simulink model "Hybrid_PID"  (R2016a)
settings: Solver=ode4  StartTime=0.0  StopTime=inf  FixedStep=ts  RelTol=1e-3
values from neighbouring files (symbols this model uses):
  db_x = 0.5    [center_and_move.m]
  db_y = 2    [center_and_move.m]
  db_z = 0.001    [center_and_move.m]
  fpos = -z_net    [center_and_move.m]
  kdx = 1.2    [center_and_move.m]
  kdy = 4    [center_and_move.m]
  kdz = 0.55    [center_and_move.m]
  kix = 3.5    [center_and_move.m]
  kiy = 1.9    [center_and_move.m]
  kiz = 10    [center_and_move.m]
  kpx = 85    [center_and_move.m]
  kpy = 485    [center_and_move.m]
  kpz = 2.5    [center_and_move.m]
  ts = 0.001    [center_and_move.m]
  tsim = 25    [center_and_move.m]
  xpos = -x_net    [center_and_move.m]    (also in genScanMatrix.m = x_net2)
  ypos = -y_net    [center_and_move.m]    (also in genScanMatrix.m = y_net)
  zpos = z_net    [genScanMatrix.m]
undefined symbols (not defined in the file or in its folder): amp, bias, f
libraries: slrtlib x11, dspswit3 x7, xpcmeasurementcomputinglib x5, simulink_extras x3, simulink x3, xpcconteclib x3, xpcutilitieslib x1, xpcrtudplib x1
settings Model: SimulationMode=external  Creator=Biorobotics  LastModifiedBy=Biorobotics
settings SolverCC: EnableConcurrentExecution=on
settings DataIOCC: SaveFormat=StructureWithTime
settings OptimizationCC: BlockReduction=off  OptimizeBlockIOStorage=off  BufferReuse=off  GlobalBufferReuse=off  ExpressionFolding=off  LocalBlockOutputs=off
settings HardwareCC: ProdBitPerPointer=32  ProdLargestAtomicFloat=None  ProdWordSize=32  ProdLongLongMode=on  ProdHWDeviceType=Generic->32-bit x86 compatible
settings RTWCC: SystemTargetFile=slrt.tlc  TemplateMakefile=slrt_default_tmf  Description=Simulink Real-Time  RTWCompilerOptimization=on

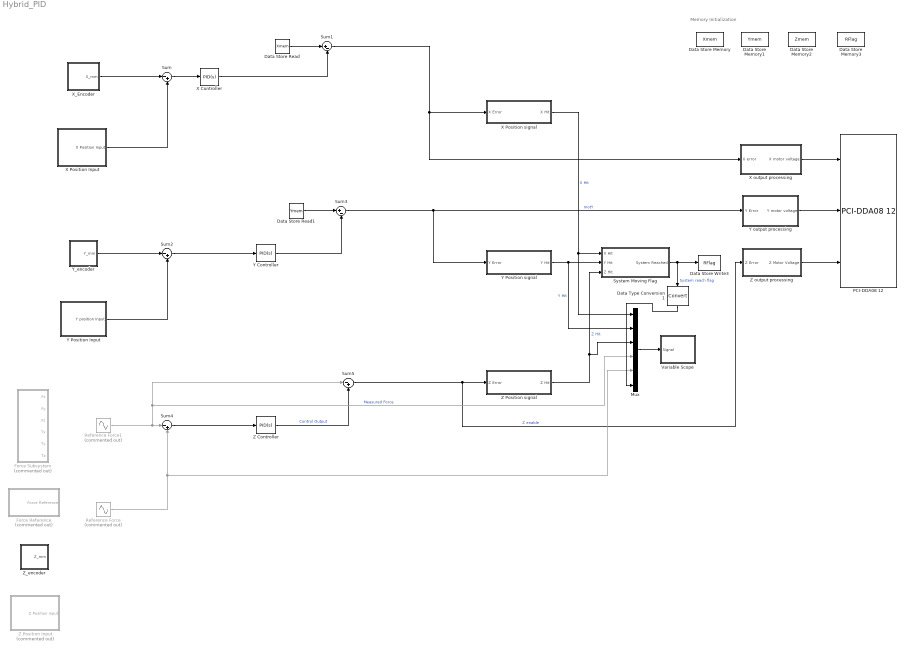
== system Hybrid_PID ==
  note: Memory Initialization
  Data Store Memory : DataStoreMemory  DataStoreName=Xmem  ReadBeforeWriteMsg=warning  WriteAfterWriteMsg=warning  WriteAfterReadMsg=warning  ShowAdditionalParam=off
  Data Store Memory1 : DataStoreMemory  DataStoreName=Ymem  ReadBeforeWriteMsg=warning  WriteAfterWriteMsg=warning  WriteAfterReadMsg=warning  ShowAdditionalParam=off
  Data Store Memory2 : DataStoreMemory  DataStoreName=Zmem  ReadBeforeWriteMsg=warning  WriteAfterWriteMsg=warning  WriteAfterReadMsg=warning  ShowAdditionalParam=off
  Data Store Memory3 : DataStoreMemory  DataStoreName=RFlag  ReadBeforeWriteMsg=warning  WriteAfterWriteMsg=warning  WriteAfterReadMsg=warning  ShowAdditionalParam=off
  Data Store Read : DataStoreRead  DataStoreName=Xmem
  Data Store Read1 : DataStoreRead  DataStoreName=Ymem
  Data Store Write3 : DataStoreWrite  DataStoreName=RFlag
  Data Type Conversion1 : DataTypeConversion
  Force Reference : Subsystem  Commented=on
  Force Subsystem : Subsystem  Commented=on
  Mux : Mux  Inputs=6
  "PCI-DDA08 12 " : xpcmeasurementcomputinglib/D//A/PCI-DDA08 12   channel=[1 2 3]  range=[-10 -10 -10]  reset=[1]  initValue=[0]  sampletime=ts  pci_dev=-1
  Reference Force : Sin  Commented=on  Amplitude=amp  Bias=bias  Frequency=f*2*pi  SampleTime=ts
  Reference Force1 : Sin  Commented=on  Amplitude=amp  Bias=bias  Frequency=f*2*pi  SampleTime=ts
  Sum{,2,4..5} (4 alike) : Sum  Inputs=|-+
  Sum1 : Sum  Inputs=|+-
  Sum3 : Sum  Inputs=|+-
  System Moving Flag : Subsystem
  Variable Scope : Subsystem
  X Controller : simulink/Continuous/PID Controller  Controller=PID  TimeDomain=Continuous-time  SampleTime=-1  IntegratorMethod=Forward Euler  FilterMethod=Forward Euler  Form=Parallel  UseFilter=on  ControllerParametersSource=internal  P=kpx  I=kix  D=kdx  N=100  InitialConditionSource=internal  InitialConditionForIntegrator=0  InitialConditionForFilter=0  ExternalReset=none  ZeroCross=off  LimitOutput=off  UpperSaturationLimit=inf  LowerSaturationLimit=-inf  LinearizeAsGain=on  AntiWindupMode=none  Kb=1  TrackingMode=off  Kt=1  PParamMin=[]  PParamMax=[]  IParamMin=[]  IParamMax=[]  DParamMin=[]  DParamMax=[]  NParamMin=[]  NParamMax=[]  KbParamMin=[]  KbParamMax=[]  KtParamMin=[]  KtParamMax=[]  POutMin=[]  POutMax=[]  IOutMin=[]  IOutMax=[]  DOutMin=[]  DOutMax=[]  NOutMin=[]  NOutMax=[]  KbOutMin=[]  KbOutMax=[]  KtOutMin=[]  KtOutMax=[]  IntegratorOutMin=[]  IntegratorOutMax=[]  FilterOutMin=[]  FilterOutMax=[]  SumOutMin=[]  SumOutMax=[]  SumI1OutMin=[]  SumI1OutMax=[]  SumI2OutMin=[]  SumI2OutMax=[]  SumI3OutMin=[]  SumI3OutMax=[]  SumDOutMin=[]  SumDOutMax=[]  SaturationOutMin=[]  SaturationOutMax=[]  IntegratorContinuousStateAttributes=''  IntegratorStateMustResolveToSignalObject=off  IntegratorRTWStateStorageClass=Auto  FilterContinuousStateAttributes=''  FilterStateMustResolveToSignalObject=off  FilterRTWStateStorageClass=Auto  DifferentiatorICPrevScaledInput=0  DifferentiatorOutMin=[]  DifferentiatorOutMax=[]
  X Position Input : Subsystem
  X Position signal : Subsystem
  X output processing : Subsystem
  X_Encoder : Subsystem
  Y Controller : simulink/Continuous/PID Controller  Controller=PID  TimeDomain=Continuous-time  SampleTime=-1  IntegratorMethod=Forward Euler  FilterMethod=Forward Euler  Form=Parallel  UseFilter=on  ControllerParametersSource=internal  P=kpy  I=kiy  D=kdy  N=100  InitialConditionSource=internal  InitialConditionForIntegrator=0  InitialConditionForFilter=0  ExternalReset=none  LimitOutput=off  UpperSaturationLimit=inf  LowerSaturationLimit=-inf  LinearizeAsGain=on  AntiWindupMode=none  Kb=1  TrackingMode=off  Kt=1  PParamMin=[]  PParamMax=[]  IParamMin=[]  IParamMax=[]  DParamMin=[]  DParamMax=[]  NParamMin=[]  NParamMax=[]  KbParamMin=[]  KbParamMax=[]  KtParamMin=[]  KtParamMax=[]  POutMin=[]  POutMax=[]  IOutMin=[]  IOutMax=[]  DOutMin=[]  DOutMax=[]  NOutMin=[]  NOutMax=[]  KbOutMin=[]  KbOutMax=[]  KtOutMin=[]  KtOutMax=[]  IntegratorOutMin=[]  IntegratorOutMax=[]  FilterOutMin=[]  FilterOutMax=[]  SumOutMin=[]  SumOutMax=[]  SumI1OutMin=[]  SumI1OutMax=[]  SumI2OutMin=[]  SumI2OutMax=[]  SumI3OutMin=[]  SumI3OutMax=[]  SumDOutMin=[]  SumDOutMax=[]  SaturationOutMin=[]  SaturationOutMax=[]  IntegratorContinuousStateAttributes=''  IntegratorStateMustResolveToSignalObject=off  IntegratorRTWStateStorageClass=Auto  FilterContinuousStateAttributes=''  FilterStateMustResolveToSignalObject=off  FilterRTWStateStorageClass=Auto  DifferentiatorICPrevScaledInput=0  DifferentiatorOutMin=[]  DifferentiatorOutMax=[]
  Y Position Input : Subsystem
  Y Position signal : Subsystem
  Y output processing : Subsystem
  "Y_encoder " : Subsystem
  Z Controller : simulink/Continuous/PID Controller  Controller=PID  TimeDomain=Continuous-time  SampleTime=-1  IntegratorMethod=Forward Euler  FilterMethod=Forward Euler  Form=Parallel  UseFilter=on  ControllerParametersSource=internal  P=kpz  I=kiz  D=kdz  N=100  InitialConditionSource=internal  InitialConditionForIntegrator=0  InitialConditionForFilter=0  ExternalReset=none  LimitOutput=off  UpperSaturationLimit=inf  LowerSaturationLimit=-inf  LinearizeAsGain=on  AntiWindupMode=none  Kb=1  TrackingMode=off  Kt=1  PParamMin=[]  PParamMax=[]  IParamMin=[]  IParamMax=[]  DParamMin=[]  DParamMax=[]  NParamMin=[]  NParamMax=[]  KbParamMin=[]  KbParamMax=[]  KtParamMin=[]  KtParamMax=[]  POutMin=[]  POutMax=[]  IOutMin=[]  IOutMax=[]  DOutMin=[]  DOutMax=[]  NOutMin=[]  NOutMax=[]  KbOutMin=[]  KbOutMax=[]  KtOutMin=[]  KtOutMax=[]  IntegratorOutMin=[]  IntegratorOutMax=[]  FilterOutMin=[]  FilterOutMax=[]  SumOutMin=[]  SumOutMax=[]  SumI1OutMin=[]  SumI1OutMax=[]  SumI2OutMin=[]  SumI2OutMax=[]  SumI3OutMin=[]  SumI3OutMax=[]  SumDOutMin=[]  SumDOutMax=[]  SaturationOutMin=[]  SaturationOutMax=[]  IntegratorContinuousStateAttributes=''  IntegratorStateMustResolveToSignalObject=off  IntegratorRTWStateStorageClass=Auto  FilterContinuousStateAttributes=''  FilterStateMustResolveToSignalObject=off  FilterRTWStateStorageClass=Auto  DifferentiatorICPrevScaledInput=0  DifferentiatorOutMin=[]  DifferentiatorOutMax=[]
  Z Position Input : Subsystem  Commented=on
  Z Position signal : Subsystem
  Z output processing : Subsystem
  Z_encoder : Subsystem
  wires:
  X_Encoder/1("X_mm ") -> Sum/1
  Sum/1 -> X Controller/1
  Y Controller/1 -> Sum3/2
  X Controller/1 -> Sum1/2
  Data Store Read1/1 -> Sum3/1
  Sum2/1 -> Y Controller/1
  Data Store Read/1 -> Sum1/1
  Z Controller/1 -> Sum5/2  "Control Output"
  Sum4/1 -> Z Controller/1
  Sum5/1 -> Z output processing/1(Z Error), Z Position signal/1(Z Error)  "Z enable"
  Z output processing/1(Z Motor Voltage) -> "PCI-DDA08 12 "/3
  Sum3/1 -> Y Position signal/1(Y Error), Y output processing/1(Y Error)  "motY"
  Y output processing/1(Y motor voltage) -> "PCI-DDA08 12 "/2
  Sum1/1 -> X output processing/1(X error), X Position signal/1(X Error)
  X output processing/1(X motor voltage) -> "PCI-DDA08 12 "/1
  X Position signal/1(X Hit) -> Mux/1, System Moving Flag/1("X Hit ")  "X Hit"
  Y Position signal/1(Y Hit) -> Mux/2, System Moving Flag/2(Y Hit)  "Y Hit"
  Z Position signal/1(Z Hit) -> System Moving Flag/3(Z Hit), Mux/3  "Z Hit"
  Mux/1 -> Variable Scope/1(Signal)
  System Moving Flag/1(System Reached) -> Data Store Write3/1, Data Type Conversion1/1  "System reach flag"
  Y Position Input/1(Y position Input) -> Sum2/2
  X Position Input/1(X Position Input) -> Sum/2
  Reference Force1/1 -> Sum5/1, Mux/4, Sum4/1  "Measured Force"
  "Y_encoder "/1(Y_mm) -> Sum2/1
  Reference Force/1 -> Mux/5, Sum4/2
  Data Type Conversion1/1 -> Mux/6

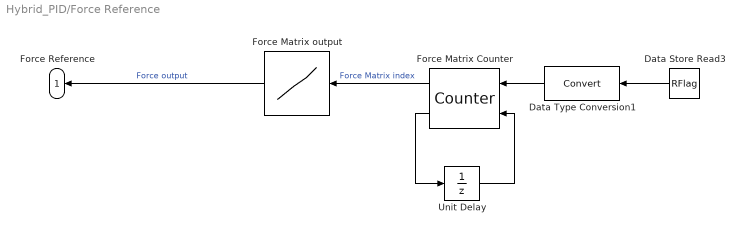
== system Hybrid_PID/Force Reference ==
  Data Store Read3 : DataStoreRead  DataStoreName=RFlag
  Data Type Conversion1 : DataTypeConversion
  Force Matrix Counter : dspswit3/Counter  Direction=Up  CountEvent=Rising edge  CounterSize=User defined  MaxCount=255  InitialCount=0  Output=Count and Hit  HitValue=20  ResetInput=on  SamplesPerFrame=1  Ts=1  CntDtype=double  HitDtype=Logical
  Force Matrix output : Lookup_n-D  NumberOfTableDimensions=1  BreakpointsSpecification=Even spacing  BreakpointsForDimension1=[0:20]  BreakpointsForDimension1FirstPoint=0  Table=fpos  InterpMethod=Flat  ExtrapMethod=Clip  UseLastTableValue=on  InternalRulePriority=Speed  RndMeth=Simplest  InputSameDT=on
  Unit Delay : UnitDelay  SampleTime=ts
  Force Reference : Outport
  wires:
  Force Matrix output/1 -> Force Reference/1  "Force output"
  Unit Delay/1 -> Force Matrix Counter/2
  Force Matrix Counter/2 -> Unit Delay/1
  Force Matrix Counter/1 -> Force Matrix output/1  "Force Matrix index"
  Data Store Read3/1 -> Data Type Conversion1/1
  Data Type Conversion1/1 -> Force Matrix Counter/1

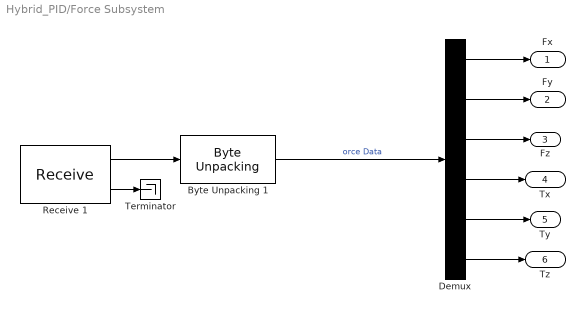
== system Hybrid_PID/Force Subsystem ==
  Byte Unpacking 1 : xpcutilitieslib/Byte Unpacking   MaskUnpackedDataTypes={'double'}  MaskUnpackedDataSizes={[6]}  MaskAlignment=1
  Demux : Demux  Outputs=6
  Receive 1 : xpcrtudplib/Legacy UDP/Receive   ipAddress=192.168.1.2  ipPort=25000  width=48  vblLen=off  sampletime=ts
  Terminator : Terminator
  Fx : Outport
  Fy : Outport  Port=2
  Fz : Outport  Port=3
  Tx : Outport  Port=4
  Ty : Outport  Port=5
  Tz : Outport  Port=6
  wires:
  Receive 1/1 -> Byte Unpacking 1/1
  Demux/3 -> Fz/1
  Byte Unpacking 1/1 -> Demux/1  "orce Data"
  Receive 1/2 -> Terminator/1
  Demux/1 -> Fx/1
  Demux/6 -> Tz/1
  Demux/5 -> Ty/1
  Demux/4 -> Tx/1
  Demux/2 -> Fy/1

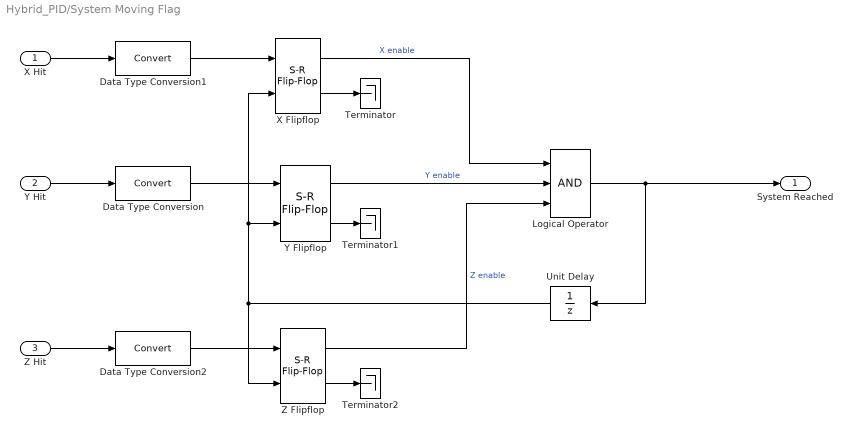
== system Hybrid_PID/System Moving Flag ==
  "X Hit " : Inport
  Y Hit : Inport  Port=2
  Z Hit : Inport  Port=3
  Data Type Conversion : DataTypeConversion
  Data Type Conversion1 : DataTypeConversion
  Data Type Conversion2 : DataTypeConversion
  Logical Operator : Logic  Inputs=3  AllPortsSameDT=off  OutDataTypeStr=boolean
  Terminator : Terminator
  Terminator1 : Terminator
  Terminator2 : Terminator
  Unit Delay : UnitDelay  SampleTime=ts
  X Flipflop : simulink_extras/Flip Flops/S-R Flip-Flop  initial_condition=0
  Y Flipflop : simulink_extras/Flip Flops/S-R Flip-Flop  initial_condition=0
  Z Flipflop : simulink_extras/Flip Flops/S-R Flip-Flop  initial_condition=0
  System Reached : Outport
  wires:
  X Flipflop/2 -> Terminator/1
  Z Flipflop/2 -> Terminator2/1
  "X Hit "/1 -> Data Type Conversion1/1
  Data Type Conversion/1 -> Y Flipflop/1
  Z Hit/1 -> Data Type Conversion2/1
  Y Hit/1 -> Data Type Conversion/1
  Data Type Conversion1/1 -> X Flipflop/1
  Data Type Conversion2/1 -> Z Flipflop/1
  Z Flipflop/1 -> Logical Operator/3  "Z enable"
  Y Flipflop/1 -> Logical Operator/2  "Y enable"
  X Flipflop/1 -> Logical Operator/1  "X enable"
  Logical Operator/1 -> System Reached/1, Unit Delay/1
  Y Flipflop/2 -> Terminator1/1
  Unit Delay/1 -> X Flipflop/2, Y Flipflop/2, Z Flipflop/2

== system Hybrid_PID/Variable Scope ==
  Signal : Inport
  Counter2 : slrtlib/Displays and Logging/Scope   scopeno=2  scopetype=Target  autostart=on  viewmode=Graphical rolling  formatstr='%15.6f'  grid=on  ylimits=[0,0]  nosamples=tsim/(5*ts)  noprepostsamples=0  interleave=1  triggermode=FreeRun  triggersignal=1  trigsignalfromport=off  triggerlevel=0.0  triggerslope=Either  triggerscope=1  triggersample=0  filename=data.dat  mode=Lazy  writesize=512  autorestart=off  dynamicfilemode=off  maxwritefilesize=512*1024^2
  Counter3 : slrtlib/Displays and Logging/Scope   scopeno=5  scopetype=File  autostart=on  viewmode=Numerical  formatstr='%15.6f'  grid=on  ylimits=[0,0]  nosamples=(10*tsim)/ts  noprepostsamples=0  interleave=1  triggermode=FreeRun  triggersignal=1  trigsignalfromport=off  triggerlevel=0.0  triggerslope=Either  triggerscope=1  triggersample=0  filename=var.dat  mode=Lazy  writesize=512  autorestart=off  dynamicfilemode=off  maxwritefilesize=512*1024^2
  wires:
  Signal/1 -> Counter2/1, Counter3/1

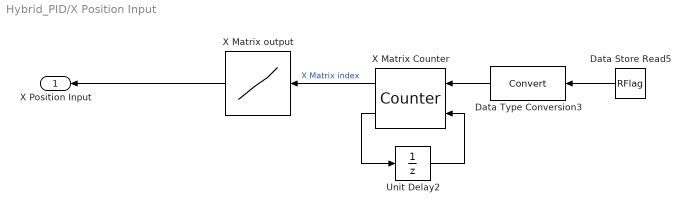
== system Hybrid_PID/X Position Input ==
  Data Store Read5 : DataStoreRead  DataStoreName=RFlag
  Data Type Conversion3 : DataTypeConversion
  Unit Delay2 : UnitDelay  SampleTime=ts
  X Matrix Counter : dspswit3/Counter  Direction=Up  CountEvent=Rising edge  CounterSize=User defined  MaxCount=255  InitialCount=0  Output=Count and Hit  HitValue=20  ResetInput=on  SamplesPerFrame=1  Ts=1  CntDtype=double  HitDtype=Logical
  X Matrix output : Lookup_n-D  NumberOfTableDimensions=1  BreakpointsSpecification=Even spacing  BreakpointsForDimension1=[0:20]  BreakpointsForDimension1FirstPoint=0  Table=xpos  InterpMethod=Flat  ExtrapMethod=Clip  UseLastTableValue=on  InternalRulePriority=Speed  RndMeth=Simplest  InputSameDT=on
  X Position Input : Outport
  wires:
  X Matrix output/1 -> X Position Input/1
  X Matrix Counter/2 -> Unit Delay2/1
  Data Type Conversion3/1 -> X Matrix Counter/1
  X Matrix Counter/1 -> X Matrix output/1  "X Matrix index"
  Data Store Read5/1 -> Data Type Conversion3/1
  Unit Delay2/1 -> X Matrix Counter/2

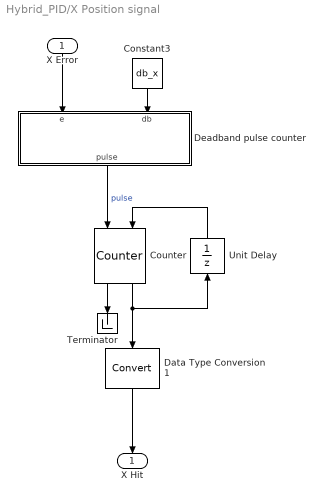
== system Hybrid_PID/X Position signal ==
  X Error : Inport
  Constant3 : Constant  Value=db_x  SampleTime=ts
  Counter : dspswit3/Counter  Direction=Up  CountEvent=Rising edge  CounterSize=User defined  MaxCount=255  InitialCount=0  Output=Count and Hit  HitValue=hitcount_x  ResetInput=on  SamplesPerFrame=1  Ts=1  CntDtype=double  HitDtype=Logical
  Data Type Conversion1 : DataTypeConversion
  Deadband pulse counter : MATLAB Function  TreatAsAtomicUnit=on
  Terminator : Terminator
  Unit Delay : UnitDelay  SampleTime=-1
  X Hit : Outport
  wires:
  Unit Delay/1 -> Counter/2
  Deadband pulse counter/1(pulse) -> Counter/1  "pulse"
  Counter/2 -> Unit Delay/1, Data Type Conversion1/1
  X Error/1 -> Deadband pulse counter/1(e)
  Data Type Conversion1/1 -> X Hit/1
  Constant3/1 -> Deadband pulse counter/2(db)
  Counter/1 -> Terminator/1

== system Hybrid_PID/X output processing ==
  X error : Inport
  Abs1 : Abs
  PCI-DDA 08 12 4 : xpcmeasurementcomputinglib/Digital Output/PCI-DDA08 12   channel=1  port=A  reset=[1]  initValue=[0]  chip=1  sampletime=ts  slot=-1
  Sign2 : Signum
  Voltage1 : Gain  Gain=3
  X motor voltage : Outport
  wires:
  Voltage1/1 -> X motor voltage/1  "x Voltage"
  Sign2/1 -> Voltage1/1, Abs1/1  "motX"
  Abs1/1 -> PCI-DDA 08 12 4/1  "X Enable"
  X error/1 -> Sign2/1

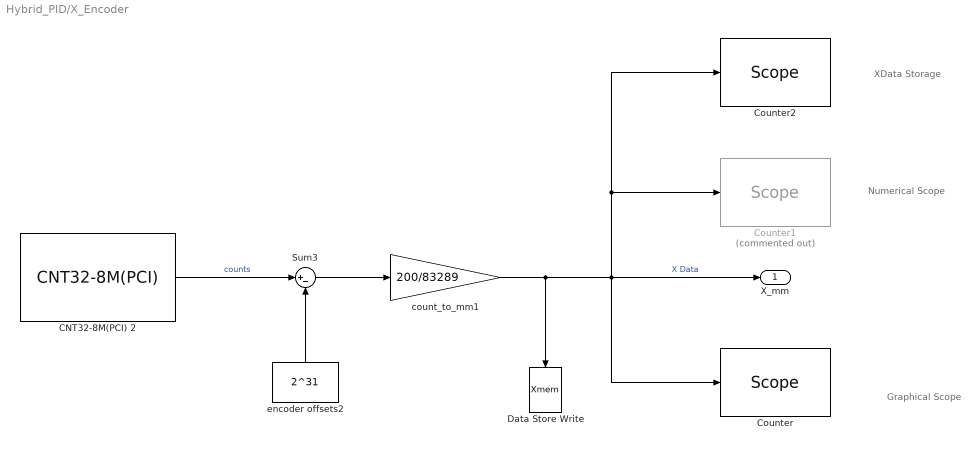
== system Hybrid_PID/X_Encoder ==
  note: Graphical Scope
  note: XData Storage
  note: Numerical Scope
  CNT32-8M(PCI) 2 : xpcconteclib/Incremental Encoder/CNT32-8M(PCI)   Channel=1  OperationMode=2-phase Input Synchronous Clear Multiply by 4  DigitalFilter=No filtering  PulseInput=TTL level input  Direction=Up in the clockwise direction/Down in the counterclockwise direction  InitialValue=2^31  LoadInitialValue=on  SampleTime=ts  PciSlot=[4 5]  StartMethod=Model Start  StopMethod=Model Terminate  ZeroClearRising=off  ZeroClearFalling=off  ZeroClearMatch0=off  ZeroClearMatch1=off  PresetRising=off  PresetFalling=off  PresetMatch0=off  PresetMatch1=off  PresetValue=0  Match0Value=0  Match1Value=0  OutputSignalMatch0=off  OutputSignalMatch1=off  OutputSignalAbnormal=off  OutputSignalDigitalFilter=off  OutputSignalAlarm=off  OneShotDuration=10 microseconds  IndexEnable=Disable  IndexLogic=Positive (Active High)  EnableDigitalInput=off  EnableDigitalOutput=off  DigitalOutputInitialValue=None  DigitalOutputFinalValue=None
  Counter : slrtlib/Displays and Logging/Scope   scopeno=3  scopetype=Target  autostart=on  viewmode=Graphical sliding  formatstr='%15.6f'  grid=on  ylimits=[0,0]  nosamples=tsim/ts  noprepostsamples=0  interleave=1  triggermode=FreeRun  triggersignal=1  trigsignalfromport=off  triggerlevel=0.0  triggerslope=Either  triggerscope=1  triggersample=0  filename=data.dat  mode=Lazy  writesize=512  autorestart=off  dynamicfilemode=off  maxwritefilesize=512*1024^2
  Counter1 : slrtlib/Displays and Logging/Scope   Commented=on  scopeno=2  scopetype=Target  autostart=on  viewmode=Numerical  formatstr='%15.6f'  grid=on  ylimits=[0,0]  nosamples=3  noprepostsamples=0  interleave=1  triggermode=FreeRun  triggersignal=1  trigsignalfromport=off  triggerlevel=0.0  triggerslope=Either  triggerscope=1  triggersample=0  filename=data.dat  mode=Lazy  writesize=512  autorestart=off  dynamicfilemode=off  maxwritefilesize=512*1024^2
  Counter2 : slrtlib/Displays and Logging/Scope   scopeno=1  scopetype=File  autostart=on  viewmode=Numerical  formatstr='%15.6f'  grid=on  ylimits=[0,0]  nosamples=(10*tsim)/ts  noprepostsamples=0  interleave=1  triggermode=FreeRun  triggersignal=1  trigsignalfromport=off  triggerlevel=0.0  triggerslope=Either  triggerscope=1  triggersample=0  filename=Xdata.dat  mode=Lazy  writesize=512  autorestart=off  dynamicfilemode=off  maxwritefilesize=512*1024^2
  Data Store Write : DataStoreWrite  DataStoreName=Xmem
  Sum3 : Sum  Inputs=|+-
  count_to_mm1 : Gain  Gain=200/83289
  encoder offsets2 : Constant  Value=2^31
  "X_mm " : Outport
  wires:
  CNT32-8M(PCI) 2/1 -> Sum3/1  "counts"
  Sum3/1 -> count_to_mm1/1
  count_to_mm1/1 -> Data Store Write/1, Counter2/1, Counter1/1, Counter/1, "X_mm "/1  "X Data"
  encoder offsets2/1 -> Sum3/2

== system Hybrid_PID/Y Position Input ==
  Data Store Read4 : DataStoreRead  DataStoreName=RFlag
  Data Type Conversion2 : DataTypeConversion
  Unit Delay1 : UnitDelay  SampleTime=ts
  Y Matrix Counter : dspswit3/Counter  Direction=Up  CountEvent=Rising edge  CounterSize=User defined  MaxCount=255  InitialCount=0  Output=Count and Hit  HitValue=20  ResetInput=on  SamplesPerFrame=1  Ts=1  CntDtype=double  HitDtype=Logical
  Y Matrix output : Lookup_n-D  NumberOfTableDimensions=1  BreakpointsSpecification=Even spacing  BreakpointsForDimension1=[0:20]  BreakpointsForDimension1FirstPoint=0  Table=ypos  InterpMethod=Flat  ExtrapMethod=Clip  UseLastTableValue=on  InternalRulePriority=Speed  RndMeth=Simplest  InputSameDT=on
  Y position Input : Outport
  wires:
  Y Matrix output/1 -> Y position Input/1
  Unit Delay1/1 -> Y Matrix Counter/2
  Data Store Read4/1 -> Data Type Conversion2/1
  Data Type Conversion2/1 -> Y Matrix Counter/1
  Y Matrix Counter/2 -> Unit Delay1/1
  Y Matrix Counter/1 -> Y Matrix output/1  "Y Matrix index"

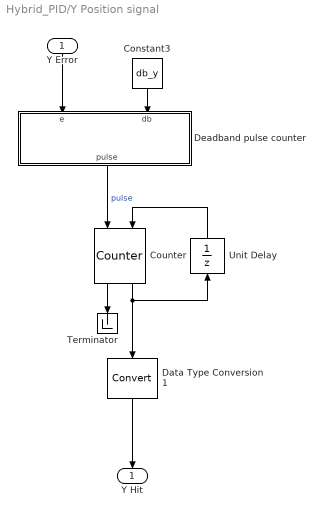
== system Hybrid_PID/Y Position signal ==
  Y Error : Inport
  Constant3 : Constant  Value=db_y  SampleTime=ts
  Counter : dspswit3/Counter  Direction=Up  CountEvent=Rising edge  CounterSize=User defined  MaxCount=255  InitialCount=0  Output=Count and Hit  HitValue=hitcount_y  ResetInput=on  SamplesPerFrame=1  Ts=1  CntDtype=double  HitDtype=Logical
  Data Type Conversion1 : DataTypeConversion
  Deadband pulse counter : MATLAB Function  TreatAsAtomicUnit=on
  Terminator : Terminator
  Unit Delay : UnitDelay  SampleTime=-1
  Y Hit : Outport
  wires:
  Unit Delay/1 -> Counter/2
  Deadband pulse counter/1(pulse) -> Counter/1  "pulse"
  Counter/2 -> Unit Delay/1, Data Type Conversion1/1
  Y Error/1 -> Deadband pulse counter/1(e)
  Data Type Conversion1/1 -> Y Hit/1
  Constant3/1 -> Deadband pulse counter/2(db)
  Counter/1 -> Terminator/1

== system Hybrid_PID/Y output processing ==
  Y Error : Inport
  Abs : Abs
  PCI-DDA 08 12 3 : xpcmeasurementcomputinglib/Digital Output/PCI-DDA08 12   channel=3  port=A  reset=[1]  initValue=[0]  chip=1  sampletime=ts  slot=-1
  Sign : Signum
  Voltage : Gain  Gain=3
  Y motor voltage : Outport
  wires:
  Abs/1 -> PCI-DDA 08 12 3/1  "Y enable"
  Voltage/1 -> Y motor voltage/1  "VoltageY"
  Sign/1 -> Voltage/1, Abs/1
  Y Error/1 -> Sign/1

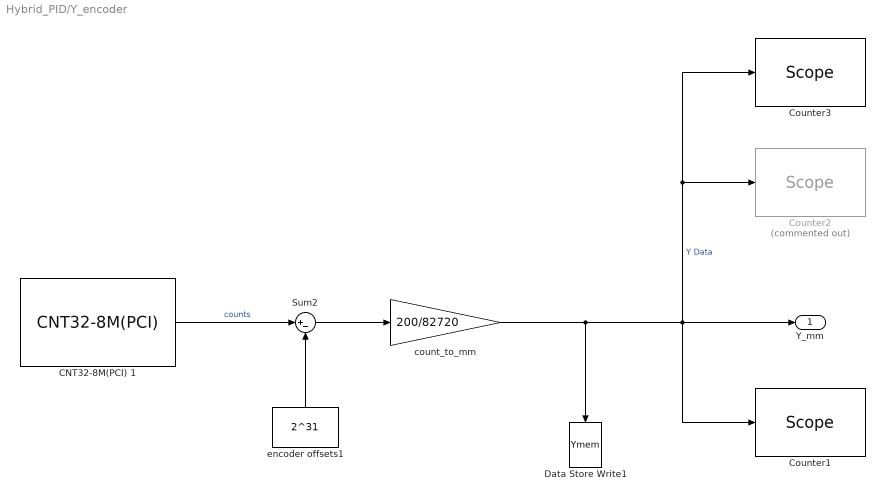
== system Hybrid_PID/Y_encoder  ==
  CNT32-8M(PCI) 1 : xpcconteclib/Incremental Encoder/CNT32-8M(PCI)   Channel=2  OperationMode=2-phase Input Synchronous Clear Multiply by 4  DigitalFilter=No filtering  PulseInput=TTL level input  Direction=Up in the clockwise direction/Down in the counterclockwise direction  InitialValue=2^31  LoadInitialValue=on  SampleTime=ts  PciSlot=[4 5]  StartMethod=Model Start  StopMethod=Model Terminate  ZeroClearRising=off  ZeroClearFalling=off  ZeroClearMatch0=off  ZeroClearMatch1=off  PresetRising=off  PresetFalling=off  PresetMatch0=off  PresetMatch1=off  PresetValue=0  Match0Value=0  Match1Value=0  OutputSignalMatch0=off  OutputSignalMatch1=off  OutputSignalAbnormal=off  OutputSignalDigitalFilter=off  OutputSignalAlarm=off  OneShotDuration=10 microseconds  IndexEnable=Disable  IndexLogic=Positive (Active High)  EnableDigitalInput=off  EnableDigitalOutput=off  DigitalOutputInitialValue=None  DigitalOutputFinalValue=None
  Counter1 : slrtlib/Displays and Logging/Scope   scopeno=6  scopetype=Target  autostart=on  viewmode=Graphical rolling  formatstr='%15.6f'  grid=on  ylimits=[0,0]  nosamples=tsim/ts  noprepostsamples=0  interleave=1  triggermode=FreeRun  triggersignal=1  trigsignalfromport=off  triggerlevel=0.0  triggerslope=Either  triggerscope=1  triggersample=0  filename=data.dat  mode=Lazy  writesize=512  autorestart=off  dynamicfilemode=off  maxwritefilesize=512*1024^2
  Counter2 : slrtlib/Displays and Logging/Scope   Commented=on  scopeno=5  scopetype=Target  autostart=on  viewmode=Numerical  formatstr='%15.6f'  grid=on  ylimits=[0,0]  nosamples=3  noprepostsamples=0  interleave=1  triggermode=FreeRun  triggersignal=1  trigsignalfromport=off  triggerlevel=0.0  triggerslope=Either  triggerscope=1  triggersample=0  filename=data.dat  mode=Lazy  writesize=512  autorestart=off  dynamicfilemode=off  maxwritefilesize=512*1024^2
  Counter3 : slrtlib/Displays and Logging/Scope   scopeno=4  scopetype=File  autostart=on  viewmode=Numerical  formatstr='%15.6f'  grid=on  ylimits=[0,0]  nosamples=(10*tsim)/ts  noprepostsamples=0  interleave=1  triggermode=FreeRun  triggersignal=1  trigsignalfromport=off  triggerlevel=0.0  triggerslope=Either  triggerscope=1  triggersample=0  filename=Ydata.dat  mode=Lazy  writesize=512  autorestart=off  dynamicfilemode=off  maxwritefilesize=512*1024^2
  Data Store Write1 : DataStoreWrite  DataStoreName=Ymem
  Sum2 : Sum  Inputs=|+-
  count_to_mm : Gain  Gain=200/82720
  encoder offsets1 : Constant  Value=2^31
  Y_mm : Outport
  wires:
  encoder offsets1/1 -> Sum2/2
  CNT32-8M(PCI) 1/1 -> Sum2/1  "counts"
  count_to_mm/1 -> Data Store Write1/1, Counter3/1, Counter2/1, Y_mm/1, Counter1/1  "Y Data"
  Sum2/1 -> count_to_mm/1

== system Hybrid_PID/Z Position Input ==
  Data Store Read3 : DataStoreRead  DataStoreName=RFlag
  Data Type Conversion1 : DataTypeConversion
  Unit Delay : UnitDelay  SampleTime=ts
  Z Matrix Counter : dspswit3/Counter  Direction=Up  CountEvent=Rising edge  CounterSize=User defined  MaxCount=255  InitialCount=0  Output=Count and Hit  HitValue=20  ResetInput=on  SamplesPerFrame=1  Ts=1  CntDtype=double  HitDtype=Logical
  Z Matrix output : Lookup_n-D  NumberOfTableDimensions=1  BreakpointsForDimension1=[0:20]  Table=zpos  InterpMethod=Flat  ExtrapMethod=Clip  UseLastTableValue=on  InternalRulePriority=Speed  RndMeth=Simplest  InputSameDT=on
  Z Position input : Outport
  wires:
  Z Matrix Counter/2 -> Unit Delay/1
  Z Matrix output/1 -> Z Position input/1  "Z Matrix output"
  Unit Delay/1 -> Z Matrix Counter/2
  Z Matrix Counter/1 -> Z Matrix output/1  "Z Matrix index"
  Data Store Read3/1 -> Data Type Conversion1/1
  Data Type Conversion1/1 -> Z Matrix Counter/1

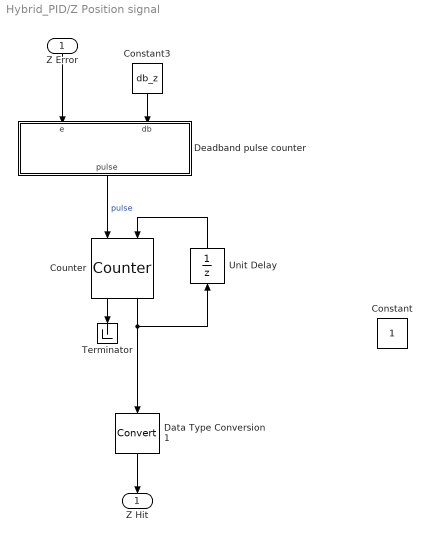
== system Hybrid_PID/Z Position signal ==
  Z Error : Inport
  Constant : Constant
  Constant3 : Constant  Value=db_z  SampleTime=ts
  Counter : dspswit3/Counter  Direction=Up  CountEvent=Rising edge  CounterSize=User defined  MaxCount=255  InitialCount=0  Output=Count and Hit  HitValue=hitcount_z  ResetInput=on  SamplesPerFrame=1  Ts=1  CntDtype=double  HitDtype=Logical
  Data Type Conversion1 : DataTypeConversion
  Deadband pulse counter : MATLAB Function  TreatAsAtomicUnit=on
  Terminator : Terminator
  Unit Delay : UnitDelay  SampleTime=ts
  Z Hit : Outport
  wires:
  Unit Delay/1 -> Counter/2
  Deadband pulse counter/1(pulse) -> Counter/1  "pulse"
  Z Error/1 -> Deadband pulse counter/1(e)
  Data Type Conversion1/1 -> Z Hit/1
  Constant3/1 -> Deadband pulse counter/2(db)
  Counter/1 -> Terminator/1
  Counter/2 -> Data Type Conversion1/1, Unit Delay/1

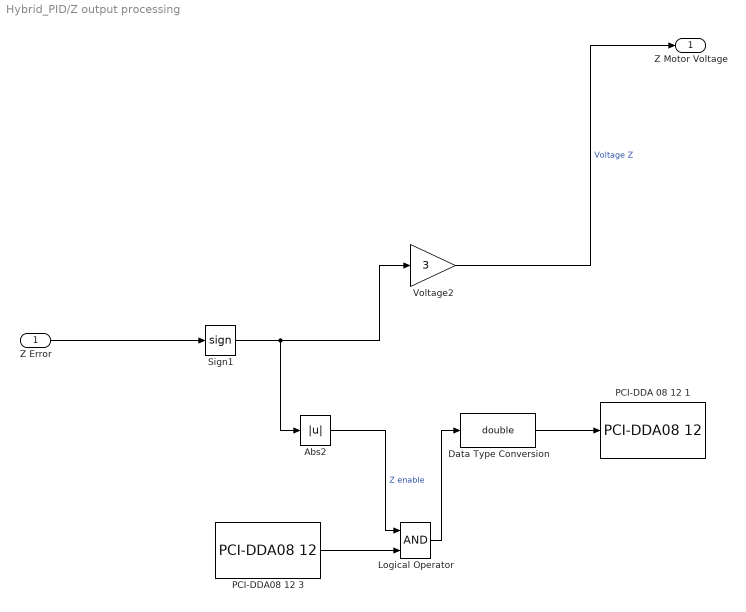
== system Hybrid_PID/Z output processing ==
  Z Error : Inport
  Abs2 : Abs
  Data Type Conversion : DataTypeConversion  OutDataTypeStr=double
  Logical Operator : Logic  AllPortsSameDT=off  OutDataTypeStr=boolean
  PCI-DDA 08 12 1 : xpcmeasurementcomputinglib/Digital Output/PCI-DDA08 12   channel=5  port=A  reset=[1]  initValue=[0]  chip=1  sampletime=ts  slot=-1
  PCI-DDA08 12 3 : xpcmeasurementcomputinglib/Digital Input/PCI-DDA08 12   channel=6  port=C  chip=2  sampletime=ts  slot=-1
  Sign1 : Signum
  Voltage2 : Gain  Gain=3
  Z Motor Voltage : Outport
  wires:
  Z Error/1 -> Sign1/1
  Sign1/1 -> Voltage2/1, Abs2/1
  Data Type Conversion/1 -> PCI-DDA 08 12 1/1
  Abs2/1 -> Logical Operator/1  "Z enable"
  Voltage2/1 -> Z Motor Voltage/1  "Voltage Z"
  PCI-DDA08 12 3/1 -> Logical Operator/2
  Logical Operator/1 -> Data Type Conversion/1

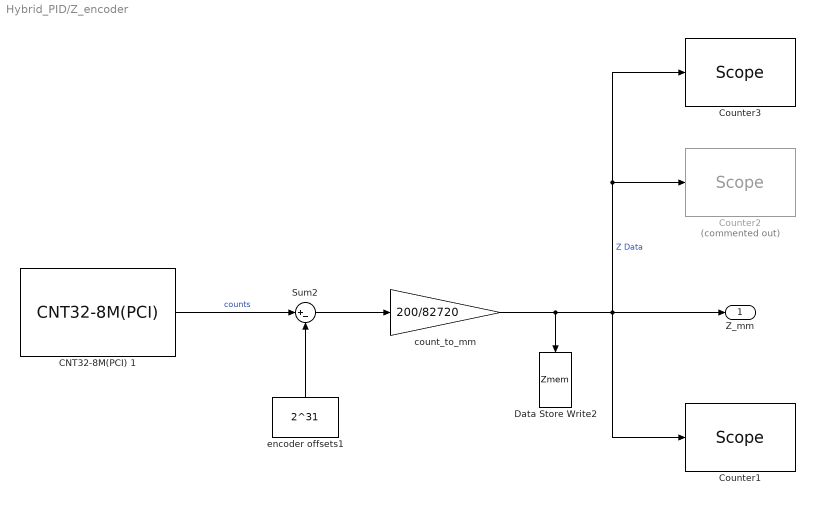
== system Hybrid_PID/Z_encoder ==
  CNT32-8M(PCI) 1 : xpcconteclib/Incremental Encoder/CNT32-8M(PCI)   Channel=4  OperationMode=2-phase Input Synchronous Clear Multiply by 4  DigitalFilter=No filtering  PulseInput=TTL level input  Direction=Up in the clockwise direction/Down in the counterclockwise direction  InitialValue=2^31  LoadInitialValue=on  SampleTime=ts  PciSlot=[4 5]  StartMethod=Model Start  StopMethod=Model Terminate  ZeroClearRising=off  ZeroClearFalling=off  ZeroClearMatch0=off  ZeroClearMatch1=off  PresetRising=off  PresetFalling=off  PresetMatch0=off  PresetMatch1=off  PresetValue=0  Match0Value=0  Match1Value=0  OutputSignalMatch0=off  OutputSignalMatch1=off  OutputSignalAbnormal=off  OutputSignalDigitalFilter=off  OutputSignalAlarm=off  OneShotDuration=10 microseconds  IndexEnable=Disable  IndexLogic=Positive (Active High)  EnableDigitalInput=off  EnableDigitalOutput=off  DigitalOutputInitialValue=None  DigitalOutputFinalValue=None
  Counter1 : slrtlib/Displays and Logging/Scope   scopeno=7  scopetype=Target  autostart=on  viewmode=Graphical rolling  formatstr='%15.6f'  grid=on  ylimits=[0,0]  nosamples=tsim/ts  noprepostsamples=0  interleave=1  triggermode=FreeRun  triggersignal=1  trigsignalfromport=off  triggerlevel=0.0  triggerslope=Either  triggerscope=1  triggersample=0  filename=data.dat  mode=Lazy  writesize=512  autorestart=off  dynamicfilemode=off  maxwritefilesize=512*1024^2
  Counter2 : slrtlib/Displays and Logging/Scope   Commented=on  scopeno=8  scopetype=Target  autostart=on  viewmode=Numerical  formatstr='%15.6f'  grid=on  ylimits=[0,0]  nosamples=3  noprepostsamples=0  interleave=1  triggermode=FreeRun  triggersignal=1  trigsignalfromport=off  triggerlevel=0.0  triggerslope=Either  triggerscope=1  triggersample=0  filename=data.dat  mode=Lazy  writesize=512  autorestart=off  dynamicfilemode=off  maxwritefilesize=512*1024^2
  Counter3 : slrtlib/Displays and Logging/Scope   scopeno=9  scopetype=File  autostart=on  viewmode=Numerical  formatstr='%15.6f'  grid=on  ylimits=[0,0]  nosamples=(10*tsim)/ts  noprepostsamples=0  interleave=1  triggermode=FreeRun  triggersignal=1  trigsignalfromport=off  triggerlevel=0.0  triggerslope=Either  triggerscope=1  triggersample=0  filename=Zdata.dat  mode=Lazy  writesize=512  autorestart=off  dynamicfilemode=off  maxwritefilesize=512*1024^2
  Data Store Write2 : DataStoreWrite  DataStoreName=Zmem
  Sum2 : Sum  Inputs=|+-
  count_to_mm : Gain  Gain=200/82720
  encoder offsets1 : Constant  Value=2^31
  Z_mm : Outport
  wires:
  encoder offsets1/1 -> Sum2/2
  CNT32-8M(PCI) 1/1 -> Sum2/1  "counts"
  count_to_mm/1 -> Data Store Write2/1, Counter1/1, Z_mm/1, Counter3/1, Counter2/1  "Z Data"
  Sum2/1 -> count_to_mm/1

== matlab function Hybrid_PID/Y Position signal/Deadband pulse counter ==
  data: e input; db input; pulse output
function pulse  = fcn(e,db)
%#codegen
if e>-db && e<db
    pulse=1;
else
    pulse=0;
end

end

== matlab function Hybrid_PID/Z Position signal/Deadband pulse counter ==
  data: e input; db input; pulse output
function pulse  = fcn(e,db)
%#codegen
if e>-db && e<db
    pulse=1;
else
    pulse=0;
end

end

== matlab function Hybrid_PID/X Position signal/Deadband pulse counter ==
  data: e input; db input; pulse output
function pulse  = fcn(e,db)
%#codegen
if e>-db && e<db
    pulse=1;
else
    pulse=0;
end

end
